simulink model "MetricsAnalyse"  (R2023a)
settings: Solver=VariableStepAuto  StartTime=0.0  StopTime=10.0  RelTol=1e-3
settings Model: Creator=19591  LastModifiedBy=19591

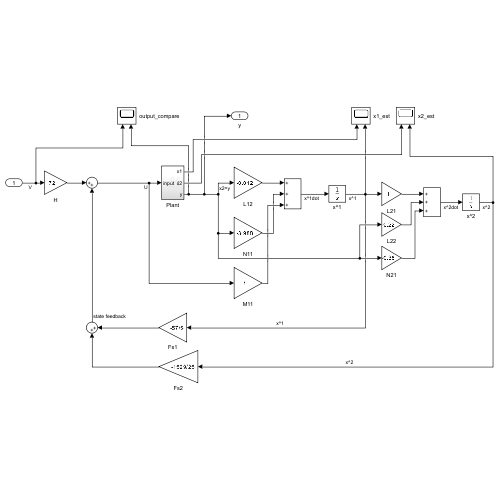
[thumbnail: Simulink's stored preview of the top-level diagram]
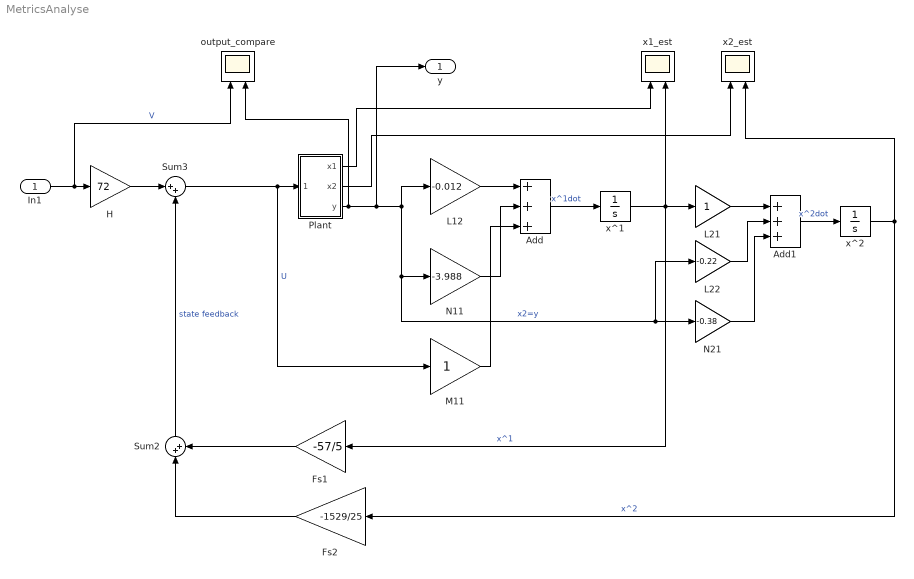
== system MetricsAnalyse ==
  In1 : Inport
  Add : Sum  Inputs=+++
  Add1 : Sum  Inputs=+++
  Fs1 : Gain  Gain=-57/5
  Fs2 : Gain  Gain=-1529/25
  H : Gain  Gain=72
  L12 : Gain  Gain=-0.012
  L21 : Gain
  L22 : Gain  Gain=-0.22
  M11 : Gain
  N11 : Gain  Gain=-3.988
  N21 : Gain  Gain=-0.38
  Plant : Subsystem
  Sum2 : Sum  Inputs=|++
  Sum3 : Sum  Inputs=|++
  output_compare : Scope  NumInputPorts=2
  x1_est : Scope  NumInputPorts=2
  x2_est : Scope  NumInputPorts=2
  x^1 : Integrator
  x^2 : Integrator
  y : Outport
  wires:
  Sum3/1 -> M11/1, Plant/1(input)  "U"
  Plant/1(x1) -> x1_est/1
  Add/1 -> x^1/1  "x^1dot"
  M11/1 -> Add/3
  N11/1 -> Add/2
  L12/1 -> Add/1
  Plant/2(x2) -> x2_est/1
  Fs1/1 -> Sum2/2
  Fs2/1 -> Sum2/1
  Add1/1 -> x^2/1  "x^2dot"
  L21/1 -> Add1/1
  N21/1 -> Add1/3
  x^2/1 -> Fs2/1, x2_est/2  "x^2"
  Plant/3(y) -> y/1, L12/1, L22/1, N21/1, N11/1, output_compare/2  "x2=y"
  L22/1 -> Add1/2
  Sum2/1 -> Sum3/2  "state feedback"
  x^1/1 -> Fs1/1, L21/1, x1_est/2  "x^1"
  In1/1 -> output_compare/1, H/1  "V"
  H/1 -> Sum3/1

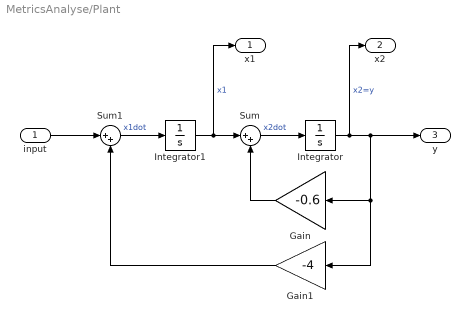
== system MetricsAnalyse/Plant ==
  input : Inport
  Gain : Gain  Gain=-0.6
  Gain1 : Gain  Gain=-4
  Integrator : Integrator
  Integrator1 : Integrator
  Sum : Sum  Inputs=|++
  Sum1 : Sum  Inputs=|++
  x1 : Outport
  x2 : Outport  Port=2
  y : Outport  Port=3
  wires:
  input/1 -> Sum1/1
  Sum1/1 -> Integrator1/1  "x1dot"
  Gain1/1 -> Sum1/2
  Sum/1 -> Integrator/1  "x2dot"
  Integrator1/1 -> x1/1, Sum/1  "x1"
  Integrator/1 -> x2/1, y/1, Gain1/1, Gain/1  "x2=y"
  Gain/1 -> Sum/2
